simulink model "Quadrotor_14_step4_disc"  (Simulink 7.6)
settings: Solver=ode45  StartTime=0.0  StopTime=200  RelTol=1e-3
undefined symbols (not defined in the file): STARMAC, uav_utilities
libraries: simulink x31, aero_sim_lib x8
(part 1 of 2)
settings Model: Creator=fluffy_bear  LastModifiedBy=jporter
settings OptimizationCC: OptimizeModelRefInitCode=on  LifeSpan=1
settings DebuggingCC: SignalRangeChecking=warning  ParameterDowncastMsg=warning  ParameterOverflowMsg=warning
settings HardwareCC: ProdLargestAtomicInteger=Long  ProdLargestAtomicFloat=Float  ProdEndianess=LittleEndian  ProdHWDeviceType=ARM Compatible->ARM 7
settings SFSimCC: SimParseCustomCode=off
settings RTWCC: SystemTargetFile=ert.tlc  GenCodeOnly=on  TemplateMakefile=ert_default_tmf  Description=Real-Time Workshop Embedded Coder  ProcessScript=ert_make_rtw_hook
settings CodeAppCC: IgnoreCustomStorageClasses=off
settings ERTTargetCC: MultiwordLength=2048  GenerateSampleERTMain=on  CombineSignalStateStructs=on  MultiInstanceERTCode=on  MultiInstanceErrorCode=Warning  ERTCustomFileTemplate=example_file_process.tlc  ConvertIfToSwitch=off

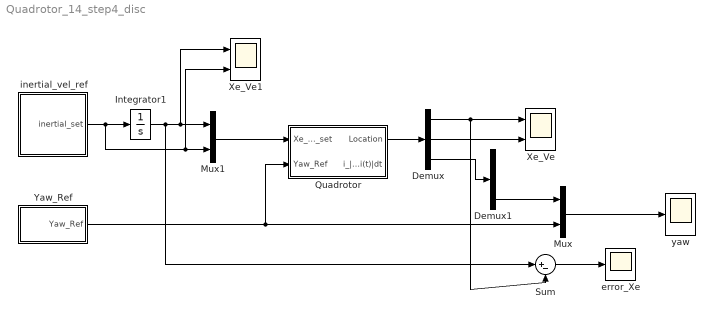
== system Quadrotor_14_step4_disc ==
  Demux : Demux  Outputs=[3,3,3]
  Demux1 : Demux  Outputs=3
  Integrator1 : Integrator
  Mux : Mux  Inputs=2
  Mux1 : Mux  Inputs=2
  Quadrotor : Subsystem  AncestorBlock=uav_utilities/STARMAC
  Sum : Sum  Inputs=|+-
  Xe_Ve : Scope  NumInputPorts=2
      settings: YMin=-25~-1  YMax=35~2.25  MaxDataPoints=100000  SampleInput=on  SampleTime=100/5000
  Xe_Ve1 : Scope  NumInputPorts=2
      settings: YMin=-100~-2  YMax=100~2  SaveName=ScopeData3  MaxDataPoints=100000  SampleInput=on  SampleTime=100/5000
  Yaw_Ref : Subsystem
  error_Xe : Scope
      settings: TimeRange=200  YMin=-1500  YMax=300  SaveName=error_data  MaxDataPoints=20000  Decimation=10  SampleInput=on  SampleTime=100/5000
  inertial_vel_ref : Subsystem
  yaw : Scope
      settings: TimeRange=2  YMin=0  YMax=115000  MaxDataPoints=100000  SampleInput=on  SampleTime=100/5000
  wires:
  inertial_vel_ref/1(inertial_set) -> Integrator1/1, Mux1/2, Xe_Ve1/2
  Yaw_Ref/1(Yaw_Ref) -> Quadrotor/2(Yaw_Ref), Mux/2
  Sum/1 -> error_Xe/1
  Quadrotor/1(Location) -> Demux/1
  Demux/1 -> Sum/2, Xe_Ve/1
  Demux/2 -> Xe_Ve/2
  Mux/1 -> yaw/1
  Demux/3 -> Demux1/1
  Demux1/3 -> Mux/1
  Integrator1/1 -> Sum/1, Mux1/1, Xe_Ve1/1
  Mux1/1 -> Quadrotor/1(Xe_Ve_set)

== system Quadrotor_14_step4_disc/Quadrotor ==
  Xe_Ve_set : Inport  PortDimensions=[6]
  Yaw_Ref : Inport  Port=2  PortDimensions=[1]
  Data Type Conversion : DataTypeConversion  OutDataTypeStr=fixdt(1,32,21)
  Data Type Conversion1 : DataTypeConversion  OutDataTypeStr=fixdt(1,32,29)
  Data Type Conversion2 : DataTypeConversion
  Demux : Demux  Outputs=[3,3]
  GPS : Subsystem
  IMU : Subsystem
  Mux : Mux  Inputs=[3 3 3]
  Rate Transition2 : RateTransition
  Subsystem : Subsystem  MinMaxOverflowLogging=MinMaxAndOverflow
  Term : Terminator
  ZOH : ZeroOrderHold  SampleTime=.01
  ZOH4 : ZeroOrderHold  SampleTime=.01
  Zero-Order Hold : ZeroOrderHold  SampleTime=.02
  dtc : DataTypeConversion
  plant_dynamics : Subsystem  AncestorBlock=aero_sim_lib/starmac_dynamics
  Location : Outport
  i_|P_i(t)|dt : Outport  Port=2
  wires:
  ZOH4/1 -> Data Type Conversion1/1
  Demux/2 -> Term/1
  Demux/1 -> ZOH/1
  Xe_Ve_set/1 -> Demux/1
  Mux/1 -> Location/1
  plant_dynamics/3(euler) -> Mux/3, IMU/1(Euler_c)  "euler"
  plant_dynamics/2(Xe) -> Mux/1, GPS/1(Xe)  "Xe"
  plant_dynamics/1(Ve) -> Mux/2, GPS/2(Ve)  "Ve"
  dtc/1 -> plant_dynamics/1(desired_motor_thrust)
  Zero-Order Hold/1 -> Rate Transition2/1
  Rate Transition2/1 -> dtc/1
  ZOH/1 -> Data Type Conversion/1
  plant_dynamics/5(omega) -> IMU/2(Omega_c)
  plant_dynamics/7(Ab) -> IMU/3(Acc_c)
  plant_dynamics/8(i_|P_i(t)|dt) -> i_|P_i(t)|dt/1
  Yaw_Ref/1 -> ZOH4/1
  IMU/1(Euler_s) -> Subsystem/1(In1)
  IMU/2(Omega_s) -> Subsystem/2(In2)
  IMU/3(Acc_s) -> Subsystem/3(In3)
  GPS/1(Latitude_s) -> Subsystem/4(In4)
  GPS/2(Longitude_s) -> Subsystem/5(In5)
  GPS/3(Height_s) -> Subsystem/6(In6)
  GPS/4(Velocity_xy_s) -> Subsystem/7(In7)
  GPS/5("dot{Height}_s") -> Subsystem/8(In8)
  Data Type Conversion/1 -> Subsystem/9(In9)
  Data Type Conversion1/1 -> Subsystem/10(In10)
  Subsystem/1(Out1) -> Data Type Conversion2/1
  Data Type Conversion2/1 -> Zero-Order Hold/1

== system Quadrotor_14_step4_disc/Yaw_Ref ==
  Signal Generator : SignalGenerator  Frequency=2*.0625*0.25
  Yaw_Ref : Outport
  wires:
  Signal Generator/1 -> Yaw_Ref/1

== system Quadrotor_14_step4_disc/inertial_vel_ref ==
  Signal Generator : SignalGenerator  Amplitude=1.8*[1 -1 -.5]  Frequency=.1*.0625*ones(3,1)
  inertial_set : Outport
  wires:
  Signal Generator/1 -> inertial_set/1

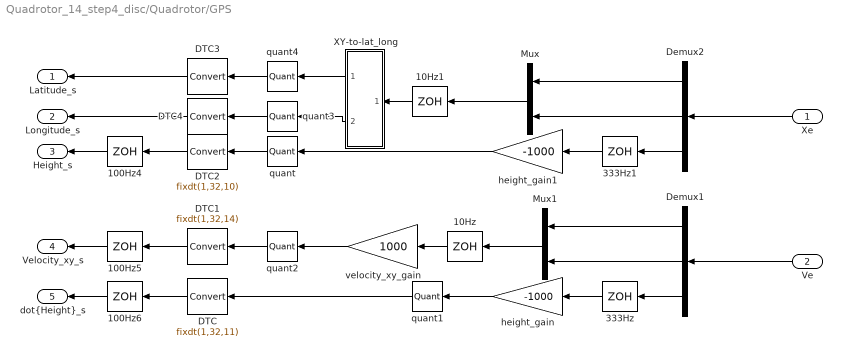
== system Quadrotor_14_step4_disc/Quadrotor/GPS ==
  Xe : Inport
  Ve : Inport  Port=2
  100Hz4 : ZeroOrderHold  SampleTime=.01
  100Hz5 : ZeroOrderHold  SampleTime=.01
  100Hz6 : ZeroOrderHold  SampleTime=.01
  10Hz : ZeroOrderHold  SampleTime=.1
  10Hz1 : ZeroOrderHold  SampleTime=.1
  333Hz : ZeroOrderHold  SampleTime=1/333
  333Hz1 : ZeroOrderHold  SampleTime=1/333
  DTC : DataTypeConversion  OutDataTypeStr=fixdt(1,32,11)
  DTC1 : DataTypeConversion  OutDataTypeStr=fixdt(1,32,14)
  DTC2 : DataTypeConversion  OutDataTypeStr=fixdt(1,32,10)
  DTC3 : DataTypeConversion
  DTC4 : DataTypeConversion
  Demux1 : Demux  Outputs=[1,1,1]
  Demux2 : Demux  Outputs=[1,1,1]
  Mux : Mux  Inputs=2
  Mux1 : Mux  Inputs=2
  XY-to-lat_long : Subsystem  mask{lat_0=36.1658333, lon_0=-86.7844444}
  height_gain : Gain  Gain=-1000  RndMeth=Round  SaturateOnIntegerOverflow=on  OutDataTypeStr=Inherit: Same as input  LockScale=on
  height_gain1 : Gain  Gain=-1000  RndMeth=Round  SaturateOnIntegerOverflow=on  OutDataTypeStr=Inherit: Same as input  LockScale=on
  quant{,1,3..4} (4 alike) : Quantizer  QuantizationInterval=1
  quant2 : Quantizer  QuantizationInterval=ones(2,1)
  velocity_xy_gain : Gain  Gain=1000  RndMeth=Round  SaturateOnIntegerOverflow=on  OutDataTypeStr=Inherit: Same as input  LockScale=on
  Latitude_s : Outport
  Longitude_s : Outport  Port=2
  Height_s : Outport  Port=3
  Velocity_xy_s : Outport  Port=4
  "dot{Height}_s" : Outport  Port=5
  wires:
  Ve/1 -> Demux1/1
  Xe/1 -> Demux2/1
  Demux1/3 -> 333Hz/1
  Demux2/3 -> 333Hz1/1
  Demux2/1 -> Mux/1
  Demux2/2 -> Mux/2
  Demux1/1 -> Mux1/1
  Demux1/2 -> Mux1/2
  333Hz1/1 -> height_gain1/1
  333Hz/1 -> height_gain/1
  Mux1/1 -> 10Hz/1
  10Hz/1 -> velocity_xy_gain/1
  height_gain1/1 -> quant/1
  height_gain/1 -> quant1/1
  quant/1 -> DTC2/1
  quant1/1 -> DTC/1
  velocity_xy_gain/1 -> quant2/1
  quant2/1 -> DTC1/1
  10Hz1/1 -> XY-to-lat_long/1(XY)
  XY-to-lat_long/1(lat) -> quant4/1
  XY-to-lat_long/2(lon) -> quant3/1
  Mux/1 -> 10Hz1/1
  DTC/1 -> 100Hz6/1
  DTC1/1 -> 100Hz5/1
  DTC2/1 -> 100Hz4/1
  DTC3/1 -> Latitude_s/1
  DTC4/1 -> Longitude_s/1
  quant3/1 -> DTC4/1
  quant4/1 -> DTC3/1
  100Hz4/1 -> Height_s/1
  100Hz5/1 -> Velocity_xy_s/1
  100Hz6/1 -> "dot{Height}_s"/1

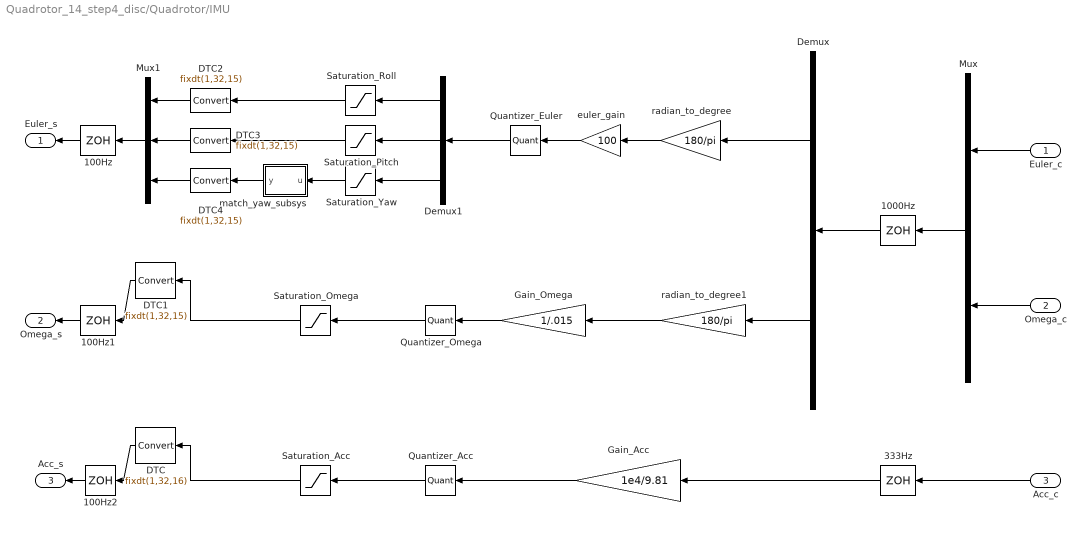
== system Quadrotor_14_step4_disc/Quadrotor/IMU ==
  Euler_c : Inport
  Omega_c : Inport  Port=2
  Acc_c : Inport  Port=3
  1000Hz : ZeroOrderHold  SampleTime=.001
  100Hz : ZeroOrderHold  SampleTime=.01
  100Hz1 : ZeroOrderHold  SampleTime=.01
  100Hz2 : ZeroOrderHold  SampleTime=.01
  333Hz : ZeroOrderHold  SampleTime=1/333
  DTC : DataTypeConversion  OutDataTypeStr=fixdt(1,32,16)
  DTC{1..4} (4 alike) : DataTypeConversion  OutDataTypeStr=fixdt(1,32,15)
  Demux : Demux  Outputs=[3,3]
  Demux1 : Demux  Outputs=[1,1,1]
  Gain_Acc : Gain  Gain=1e4/9.81
  Gain_Omega : Gain  Gain=1/.015
  Mux : Mux  Inputs=[3,3]
  Mux1 : Mux  Inputs=[1,1,1]
  Quantizer_Acc : Quantizer  QuantizationInterval=ones(3,1)
  Quantizer_Euler : Quantizer  QuantizationInterval=ones(3,1)
  Quantizer_Omega : Quantizer  QuantizationInterval=ones(3,1)
  Saturation_Acc : Saturate  UpperLimit=30000  LowerLimit=-30000  RndMeth=Round
      settings: LockScale=on
  Saturation_Omega : Saturate  UpperLimit=((2^15)-1) * ones(3,1)  LowerLimit=-(2^15) * ones(3,1)  OutDataTypeStr=Inherit: Inherit via back propagation  RndMeth=Round
      settings: LockScale=on
  Saturation_Pitch : Saturate  UpperLimit=90*100  LowerLimit=-90*100  RndMeth=Round
      settings: LockScale=on
  Saturation_Roll : Saturate  UpperLimit=90*100  LowerLimit=-90*100  RndMeth=Round
      settings: LockScale=on
  Saturation_Yaw : Saturate  UpperLimit=180*100  LowerLimit=-180*100  RndMeth=Round
      settings: LockScale=on
  euler_gain : Gain  Gain=100
  match_yaw_subsys : Subsystem
  radian_to_degree : Gain  Gain=180/pi
  radian_to_degree1 : Gain  Gain=180/pi
  Euler_s : Outport  LockScale=on
  Omega_s : Outport  Port=2  LockScale=on
  Acc_s : Outport  Port=3  LockScale=on
  wires:
  Mux/1 -> 1000Hz/1
  Euler_c/1 -> Mux/1
  1000Hz/1 -> Demux/1
  Gain_Acc/1 -> Quantizer_Acc/1
  Omega_c/1 -> Mux/2
  333Hz/1 -> Gain_Acc/1
  Saturation_Acc/1 -> DTC/1
  Saturation_Omega/1 -> DTC1/1
  Demux1/1 -> Saturation_Roll/1
  Saturation_Roll/1 -> DTC2/1
  Mux1/1 -> 100Hz/1
  Demux1/2 -> Saturation_Pitch/1
  Saturation_Pitch/1 -> DTC3/1
  Demux1/3 -> Saturation_Yaw/1
  Gain_Omega/1 -> Quantizer_Omega/1
  Demux/1 -> radian_to_degree/1
  radian_to_degree/1 -> euler_gain/1
  Demux/2 -> radian_to_degree1/1
  euler_gain/1 -> Quantizer_Euler/1
  Quantizer_Euler/1 -> Demux1/1
  radian_to_degree1/1 -> Gain_Omega/1
  Quantizer_Omega/1 -> Saturation_Omega/1
  Acc_c/1 -> 333Hz/1
  Quantizer_Acc/1 -> Saturation_Acc/1
  DTC/1 -> 100Hz2/1
  DTC1/1 -> 100Hz1/1
  100Hz/1 -> Euler_s/1
  100Hz1/1 -> Omega_s/1
  100Hz2/1 -> Acc_s/1
  match_yaw_subsys/1(y) -> DTC4/1
  Saturation_Yaw/1 -> match_yaw_subsys/1(u)
  DTC2/1 -> Mux1/1
  DTC3/1 -> Mux1/2
  DTC4/1 -> Mux1/3

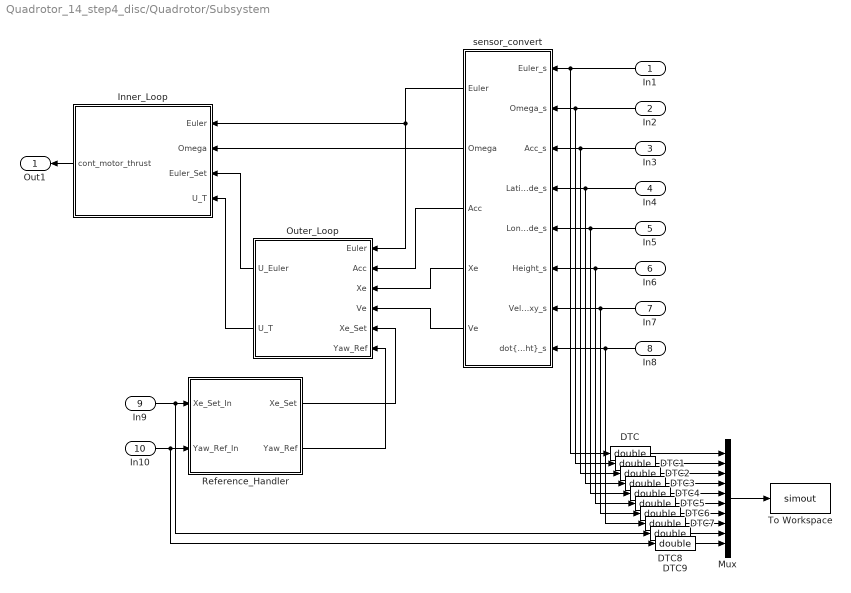
== system Quadrotor_14_step4_disc/Quadrotor/Subsystem ==
  In1 : Inport  OutMin=-36000  OutMax=36000  OutDataTypeStr=fixdt(1,32,15)
  In2 : Inport  Port=2  OutMin=-(2^15)  OutMax=2^15  OutDataTypeStr=fixdt(1,32,15)
  In3 : Inport  Port=3  OutMin=-30000  OutMax=30000  OutDataTypeStr=fixdt(1,32,16)
  In4 : Inport  Port=4  OutMin=-90*1e7  OutMax=90*1e7  OutDataTypeStr=fixdt(1,32,0)
  In5 : Inport  Port=5  OutMin=-180*1e7  OutMax=180*1e7  OutDataTypeStr=fixdt(1,32,0)
  In6 : Inport  Port=6  OutMin=-2000*1000  OutMax=2000*1000  OutDataTypeStr=fixdt(1,32,10)
  In7 : Inport  Port=7  OutMin=-100*1000  OutMax=100*1000  OutDataTypeStr=fixdt(1,32,14)
  In8 : Inport  Port=8  OutMin=-100*1000  OutMax=1000*1000  OutDataTypeStr=fixdt(1,32,11)
  In9 : Inport  Port=9  OutMin=-1000  OutMax=1000  OutDataTypeStr=fixdt(1,32,21)
  In10 : Inport  Port=10  OutMin=-pi  OutMax=pi  OutDataTypeStr=fixdt(1,32,29)
  DTC{,1..9} (10 alike) : DataTypeConversion  OutDataTypeStr=double
  Inner_Loop : Subsystem
  Mux : Mux  Inputs=10
  Outer_Loop : Subsystem
  Reference_Handler : Subsystem
  To Workspace : ToWorkspace  VariableName=simout  SampleTime=-1  SaveFormat=Structure
  sensor_convert : Subsystem
  Out1 : Outport
  wires:
  Outer_Loop/1(U_Euler) -> Inner_Loop/3(Euler_Set)
  Outer_Loop/2(U_T) -> Inner_Loop/4(U_T)
  sensor_convert/1(Euler) -> Inner_Loop/1(Euler), Outer_Loop/1(Euler)
  sensor_convert/2(Omega) -> Inner_Loop/2(Omega)
  sensor_convert/3(Acc) -> Outer_Loop/2(Acc)
  sensor_convert/4(Xe) -> Outer_Loop/3(Xe)
  sensor_convert/5(Ve) -> Outer_Loop/4(Ve)
  Reference_Handler/1(Xe_Set) -> Outer_Loop/5(Xe_Set)
  Reference_Handler/2(Yaw_Ref) -> Outer_Loop/6(Yaw_Ref)
  In1/1 -> sensor_convert/1(Euler_s), DTC/1
  In2/1 -> sensor_convert/2(Omega_s), DTC1/1
  In3/1 -> sensor_convert/3(Acc_s), DTC2/1
  Inner_Loop/1(cont_motor_thrust) -> Out1/1
  In4/1 -> sensor_convert/4(Latitude_s), DTC3/1
  In5/1 -> sensor_convert/5(Longitude_s), DTC4/1
  In6/1 -> sensor_convert/6(Height_s), DTC5/1
  In7/1 -> sensor_convert/7(Velocity_xy_s), DTC6/1
  In8/1 -> sensor_convert/8("dot{Height}_s"), DTC7/1
  In9/1 -> Reference_Handler/1(Xe_Set_In), DTC8/1
  In10/1 -> Reference_Handler/2(Yaw_Ref_In), DTC9/1
  Mux/1 -> To Workspace/1
  DTC/1 -> Mux/1
  DTC1/1 -> Mux/2
  DTC2/1 -> Mux/3
  DTC3/1 -> Mux/4
  DTC4/1 -> Mux/5
  DTC5/1 -> Mux/6
  DTC6/1 -> Mux/7
  DTC7/1 -> Mux/8
  DTC8/1 -> Mux/9
  DTC9/1 -> Mux/10

== system Quadrotor_14_step4_disc/Quadrotor/plant_dynamics ==
  desired_motor_thrust : Inport
  6DOF_Euler_Angles : Subsystem  AncestorBlock=aero_sim_lib/6DOF (Euler Angles)_CMU  mask{XYZe_0=[0.01;0.01;0], Vb_0=[0;0;0], euler_0=[0;0;0], omega_0=[0;0;0], M=1.8623, I=diag([0.02759 0.02771 0.04806])}
      mask prompts: XYZe_0 "Initial position in inertial axes [Xe,Ye,Ze]:"; Vb_0 "Initial velocity in body axes [U,v,w]:"; euler_0 "Initial Euler orientation [roll, pitch, yaw]=[phi,theta,psi]:"; omega_0 "Initial body rotation rates [p,q,r]=omega:"; M "Initial mass:"; I "Inertial:"
  Abs : Abs
  Dot Product : DotProduct  InputSameDT=on  OutDataTypeStr=Inherit: Inherit via internal rule
  Integrator : Integrator
  Product : Product  Multiplication=Matrix(*)  RndMeth=Zero
  Product1 : Product  Multiplication=Matrix(*)  RndMeth=Zero
  Sum : Sum  Inputs=|+++
  Sum1 : Sum  Inputs=|+-
  Viscous Drag : Gain  Gain=-.1
  gravity_effects : Constant  Value=1.8623*[0;0;9.8]
  gravity_effects1 : Constant  Value=zeros(3,1)
  starmac_blade_flapping_effects : Subsystem  AncestorBlock=aero_sim_lib/starmac_blade_flapping_effects
  starmac_motor_dynamics : Subsystem  AncestorBlock=aero_sim_lib/starmac_motor_dynamics  mask{tau_motor=.1, T_nom=1.8263*9.8/4, thrust_max=9.8, thrust_min=0, motor_lag_enable=on, motor_variance=.01*(.05*9.8/4)^2, Ts=1/76}
      mask prompts: tau_motor "tau_motor (seconds):"; T_nom "nominal thrust (N):"; thrust_max "maximum thrust (N):"; thrust_min "minimum thrust (N):"; motor_lag_enable "Motor Lag Enabled:"; motor_variance "Motor Variance [motor_variance]:"; Ts "Motor Update Rate (seconds):"
  Ve : Outport
  Xe : Outport  Port=2
  euler : Outport  Port=3
  DCM : Outport  Port=4
  omega : Outport  Port=5
  domega/dt : Outport  Port=6
  Ab : Outport  Port=7
  i_|P_i(t)|dt : Outport  Port=8
  wires:
  desired_motor_thrust/1 -> starmac_motor_dynamics/1(desired_motor_thrust)
  starmac_blade_flapping_effects/1(body_forces) -> Sum/2, Dot Product/1
  starmac_blade_flapping_effects/2(body_moments) -> 6DOF_Euler_Angles/2(M_xyz(Nm))
  Viscous Drag/1 -> Sum/3
  6DOF_Euler_Angles/5(Vb) -> Sum1/1, Dot Product/2
  Product1/1 -> Sum1/2
  Sum1/1 -> Viscous Drag/1, starmac_blade_flapping_effects/2(v_body_relative)
  gravity_effects/1 -> Product/2
  6DOF_Euler_Angles/4(DCM) -> Product1/1, Product/1, DCM/1
  Sum/1 -> 6DOF_Euler_Angles/1(F_xyz(N))
  Product/1 -> Sum/1
  starmac_motor_dynamics/1(motor_thrust) -> starmac_blade_flapping_effects/1(motor_thrusts)
  6DOF_Euler_Angles/1(Ve) -> Ve/1
  6DOF_Euler_Angles/2(Xe) -> Xe/1
  6DOF_Euler_Angles/3(euler) -> euler/1
  6DOF_Euler_Angles/6(omega) -> omega/1
  6DOF_Euler_Angles/7(domega/dt) -> domega/dt/1
  6DOF_Euler_Angles/8(Ab) -> Ab/1
  Integrator/1 -> i_|P_i(t)|dt/1
  Dot Product/1 -> Abs/1
  Abs/1 -> Integrator/1
  gravity_effects1/1 -> Product1/2

== system Quadrotor_14_step4_disc/Quadrotor/GPS/XY-to-lat_long ==
  XY : Inport
  XY-to-lat_long : Stateflow chart  TreatAsAtomicUnit=on
  lat : Outport
  lon : Outport  Port=2
  wires:
  XY-to-lat_long/1(lat) -> lat/1
  XY/1 -> XY-to-lat_long/1(XY)
  XY-to-lat_long/2(lon) -> lon/1

== system Quadrotor_14_step4_disc/Quadrotor/IMU/match_yaw_subsys ==
  u : Inport
  Constant : Constant  Value=360
  Sum : Sum  Inputs=++|
  Switch : Switch
  euler_gain1 : Gain  Gain=100
  y : Outport
  wires:
  u/1 -> Switch/2, Sum/1, Switch/1
  Constant/1 -> euler_gain1/1
  euler_gain1/1 -> Sum/2
  Sum/1 -> Switch/3
  Switch/1 -> y/1

== system Quadrotor_14_step4_disc/Quadrotor/Subsystem/Inner_Loop ==
  Euler : Inport
  Omega : Inport  Port=2
  Euler_Set : Inport  Port=3
  U_T : Inport  Port=4
  DTC{,1..3} (4 alike) : DataTypeConversion
  euler_controller : Subsystem  mask{K=1, K_e=7.5/.65, K_o=.5}
      mask prompts: K "Loop Gain [K]:"; K_e "Euler Gain [K_e]:"; K_o "Omega Gain [K_o]:"
  lead_motor : Subsystem  mask{tau_motor=.10, t_s=.01}
      mask init:
      | Hs=tf([tau_motor 1],[t_s/pi 1]);
      | Hz=ipesh_transform(Hs,t_s);
  thrust_limit : Saturate  UpperLimit=10*ones(4,1)  LowerLimit=0*ones(4,1)  OutDataTypeStr=fixdt(1,32,27)
  u_T_u_torque_motor_thrust : Subsystem  mask{dx=.3048, K_torque=.47}
      mask prompts: dx "X distance of motor from CG [dx](meters):"; K_torque "Ktorque [K_torque]:"
      mask init:
      | M=[0 -dx 0 dx;
      |    dx 0 -dx 0;
      |    -K_torque K_torque -K_torque K_torque;
      |    1 1 1 1];
      | Mi=inv(M);
  cont_motor_thrust : Outport
  wires:
  Euler_Set/1 -> DTC/1
  U_T/1 -> DTC3/1
  euler_controller/1(u_torque) -> u_T_u_torque_motor_thrust/1(u_torque)
  thrust_limit/1 -> cont_motor_thrust/1
  u_T_u_torque_motor_thrust/1(cont_motor_thrust) -> lead_motor/1(thrust_in)
  lead_motor/1(thrust_out) -> thrust_limit/1
  Euler/1 -> DTC1/1
  Omega/1 -> DTC2/1
  DTC/1 -> euler_controller/1(euler_set)
  DTC1/1 -> euler_controller/2(euler)
  DTC2/1 -> euler_controller/3(omega)
  DTC3/1 -> u_T_u_torque_motor_thrust/2(u_T)

== system Quadrotor_14_step4_disc/Quadrotor/Subsystem/Outer_Loop ==
  Euler : Inport  PortDimensions=[3]
  Acc : Inport  Port=2  PortDimensions=[3]
  Xe : Inport  Port=3  PortDimensions=[3]
  Ve : Inport  Port=4  PortDimensions=[3]
  Xe_Set : Inport  Port=5  PortDimensions=[3]
  Yaw_Ref : Inport  Port=6  PortDimensions=[1]
  DTC : DataTypeConversion
  DTC1 : DataTypeConversion  OutDataTypeStr=fixdt(1,32,26)
  DTC2 : DataTypeConversion  OutDataTypeStr=fixdt(1,32,27)
  DTC3 : DataTypeConversion  OutDataTypeStr=fixdt(1,32,20)
  DTC4 : DataTypeConversion
  DTC5 : DataTypeConversion
  Demux : Demux  Outputs=3
  body_to_inertial : Subsystem
  inertial_pos_controller : Subsystem
  rate_limiter_quant : Subsystem  mask{wn=2*pi, zeta=0.9, Vmax=2, T=0.01}
      mask prompts: wn "omega_n"; Vmax "Max velocity"; T "Sample time"
      mask init:
      | Hs=tf([wn^2],[1,2*zeta*wn,wn^2]);
      | Hz=ipesh_transform(Hs,T);
  sensor_fusion : Subsystem  mask{tau=.1, Ts=.01, Ts_gps=.1}
      mask prompts: tau "low-pass time constant (sec) [tau]"; Ts "Sample time [Ts]"; Ts_gps "GPS Sample Time [Ts_gps]"
  U_Euler : Outport  PortDimensions=[3]
  U_T : Outport  Port=2  PortDimensions=[1]
  wires:
  Xe_Set/1 -> DTC3/1
  inertial_pos_controller/1(u_T) -> U_T/1
  inertial_pos_controller/2(u_euler) -> U_Euler/1
  Euler/1 -> DTC2/1
  Acc/1 -> DTC1/1
  sensor_fusion/1(Xe) -> inertial_pos_controller/2(Xe)
  sensor_fusion/2(Ve) -> inertial_pos_controller/3(Ve)
  body_to_inertial/1(Xe) -> sensor_fusion/1(Xe_f)
  body_to_inertial/2(Ve) -> sensor_fusion/2(Ve_f)
  Xe/1 -> DTC4/1
  Ve/1 -> DTC5/1
  rate_limiter_quant/1(Xr_set) -> inertial_pos_controller/1(Xe_set)
  Demux/3 -> inertial_pos_controller/4(Yaw_actual)
  Yaw_Ref/1 -> DTC/1
  DTC/1 -> inertial_pos_controller/5(Yaw_set)
  DTC1/1 -> body_to_inertial/2(Ab)
  DTC2/1 -> body_to_inertial/1(euler), Demux/1
  DTC3/1 -> rate_limiter_quant/1(Xe_set)
  DTC4/1 -> sensor_fusion/3(Xe_s)
  DTC5/1 -> sensor_fusion/4(Ve_s)

== system Quadrotor_14_step4_disc/Quadrotor/Subsystem/Reference_Handler ==
  Xe_Set_In : Inport
  Yaw_Ref_In : Inport  Port=2
  DTC : DataTypeConversion
  DTC1 : DataTypeConversion
  Gain : Gain  ParamMin=1  ParamMax=1  OutDataTypeStr=fixdt(1,32,21)
  Gain1 : Gain  ParamMin=1  ParamMax=1  OutDataTypeStr=fixdt(1,32,29)
  Xe_Set : Outport
  Yaw_Ref : Outport  Port=2
  wires:
  Xe_Set_In/1 -> Gain/1
  Yaw_Ref_In/1 -> Gain1/1
  Gain1/1 -> DTC1/1
  Gain/1 -> DTC/1
  DTC/1 -> Xe_Set/1
  DTC1/1 -> Yaw_Ref/1

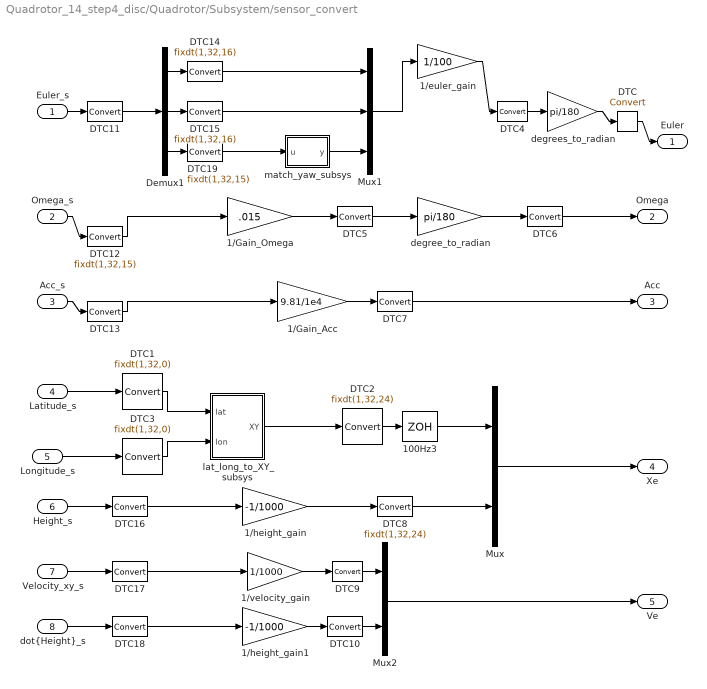
== system Quadrotor_14_step4_disc/Quadrotor/Subsystem/sensor_convert ==
  Euler_s : Inport
  Omega_s : Inport  Port=2
  Acc_s : Inport  Port=3
  Latitude_s : Inport  Port=4
  Longitude_s : Inport  Port=5
  Height_s : Inport  Port=6
  Velocity_xy_s : Inport  Port=7
  "dot{Height}_s" : Inport  Port=8
  1/Gain_Acc : Gain  Gain=9.81/1e4  ParamMin=9.81/1e4  ParamMax=9.81/1e4  OutDataTypeStr=fixdt(1,32,26)
  1/Gain_Omega : Gain  Gain=.015  ParamMin=.015  ParamMax=.015  OutDataTypeStr=fixdt(1,32,22)
  1/euler_gain : Gain  Gain=1/100  ParamMin=1/100  ParamMax=1/100  OutDataTypeStr=fixdt(1,32,23)
  1/height_gain : Gain  Gain=-1/1000  ParamMin=-1/1000  ParamMax=-1/1000  OutDataTypeStr=fixdt(1,32,25)
  1/height_gain1 : Gain  Gain=-1/1000  ParamMin=-1/1000  ParamMax=-1/1000  OutDataTypeStr=fixdt(1,32,31)
  1/velocity_gain : Gain  Gain=1/1000  ParamMin=1/1000  ParamMax=1/1000  OutDataTypeStr=fixdt(1,32,30)
  100Hz3 : ZeroOrderHold  SampleTime=.01
  DTC{,4..7,9..11,13,16..18} (12 alike) : DataTypeConversion
  DTC1 : DataTypeConversion  OutDataTypeStr=fixdt(1,32,0)
  DTC12 : DataTypeConversion  OutDataTypeStr=fixdt(1,32,15)
  DTC14 : DataTypeConversion  OutMin=-9000  OutMax=9000  OutDataTypeStr=fixdt(1,32,16)
  DTC15 : DataTypeConversion  OutMin=-9000  OutMax=9000  OutDataTypeStr=fixdt(1,32,16)
  DTC19 : DataTypeConversion  OutMin=0  OutMax=36000  OutDataTypeStr=fixdt(1,32,15)
  DTC2 : DataTypeConversion  OutDataTypeStr=fixdt(1,32,24)
  DTC3 : DataTypeConversion  OutDataTypeStr=fixdt(1,32,0)
  DTC8 : DataTypeConversion  OutDataTypeStr=fixdt(1,32,24)
  Demux1 : Demux  Outputs=3
  Mux : Mux  Inputs=[2,1]
  Mux1 : Mux  Inputs=3
  Mux2 : Mux  Inputs=[2,1]
  degree_to_radian : Gain  Gain=pi/180  ParamMin=pi/180  ParamMax=pi/180  OutDataTypeStr=fixdt(1,32,27)
  degrees_to_radian : Gain  Gain=pi/180  ParamMin=pi/180  ParamMax=pi/180  OutDataTypeStr=fixdt(1,32,27)
  lat_long_to_XY_subsys : Subsystem
  match_yaw_subsys : Subsystem
  Euler : Outport
  Omega : Outport  Port=2
  Acc : Outport  Port=3
  Xe : Outport  Port=4
  Ve : Outport  Port=5
  wires:
  Omega_s/1 -> DTC12/1
  1/Gain_Omega/1 -> DTC5/1
  1/Gain_Acc/1 -> DTC7/1
  Acc_s/1 -> DTC13/1
  degree_to_radian/1 -> DTC6/1
  Euler_s/1 -> DTC11/1
  Mux1/1 -> 1/euler_gain/1
  degrees_to_radian/1 -> DTC/1
  1/euler_gain/1 -> DTC4/1
  Demux1/1 -> DTC14/1
  Demux1/2 -> DTC15/1
  match_yaw_subsys/1(y) -> Mux1/3
  Demux1/3 -> DTC19/1
  Velocity_xy_s/1 -> DTC17/1
  Height_s/1 -> DTC16/1
  1/height_gain/1 -> DTC8/1
  Latitude_s/1 -> DTC1/1
  Longitude_s/1 -> DTC3/1
  lat_long_to_XY_subsys/1(XY) -> DTC2/1
  100Hz3/1 -> Mux/1
  Mux/1 -> Xe/1
  "dot{Height}_s"/1 -> DTC18/1
  1/height_gain1/1 -> DTC10/1
  Mux2/1 -> Ve/1
  DTC2/1 -> 100Hz3/1
  1/velocity_gain/1 -> DTC9/1
  DTC1/1 -> lat_long_to_XY_subsys/1(lat)
  DTC3/1 -> lat_long_to_XY_subsys/2(lon)
  DTC/1 -> Euler/1
  DTC4/1 -> degrees_to_radian/1
  DTC5/1 -> degree_to_radian/1
  DTC6/1 -> Omega/1
  DTC7/1 -> Acc/1
  DTC8/1 -> Mux/2
  DTC9/1 -> Mux2/1
  DTC10/1 -> Mux2/2
  DTC11/1 -> Demux1/1
  DTC12/1 -> 1/Gain_Omega/1
  DTC13/1 -> 1/Gain_Acc/1
  DTC16/1 -> 1/height_gain/1
  DTC17/1 -> 1/velocity_gain/1
  DTC18/1 -> 1/height_gain1/1
  DTC14/1 -> Mux1/1
  DTC15/1 -> Mux1/2
  DTC19/1 -> match_yaw_subsys/1(u)

== system Quadrotor_14_step4_disc/Quadrotor/plant_dynamics/6DOF_Euler_Angles ==
  note: This subsystem models a 6 degree of freedom (6DOF) system in Euler angles.
      | A Direct Cosine Matrix (DCM) is produced to allow for easy transformations to
      | and from the reference frame of the body.  Enter appropriate Parameters in the dialog menu.
      | Follows Euler Angle Sequence (1,2,3), see Section 5.6, Representing Attitude: Euler Angles, Unit
      | Quaternions, and Rotation by James Diebel.  Interface matches that from the Aerospace Toolbox
      | for non variable mass (6DoF EoM (Body Axis) for Euler Angles).
      |
      | J. Kapinski
      | Carnegia Mellon University
      | 7/2007
      | Revised:
      | Nicholas Kottenstette, ISIS, 8/2008
  note: 6 DOF System Model
  F_xyz(N) : Inport
  M_xyz(Nm) : Inport  Port=2  PortDimensions=3
  body_euler_to_earth : aero_sim_lib/body_euler_to_earth  SystemSampleTime=-1  XYZe_0=XYZe_0
  continuous_body_dynamics : aero_sim_lib/continuous_body_dynamics  SystemSampleTime=-1  M=M  Vb_0=Vb_0
  continuous_inertia_body_dynamics : aero_sim_lib/continuous_inertia_body_dynamics  SystemSampleTime=-1  I=I  omega_0=omega_0
  omega_to_euler : aero_sim_lib/omega_to_euler  SystemSampleTime=-1  euler_0=euler_0
  Ve : Outport
  Xe : Outport  Port=2
  euler : Outport  Port=3
  DCM : Outport  Port=4
  Vb : Outport  Port=5
  omega : Outport  Port=6
  domega/dt : Outport  Port=7
  Ab : Outport  Port=8
  wires:
  body_euler_to_earth/3 -> Xe/1
  body_euler_to_earth/2 -> DCM/1
  body_euler_to_earth/1 -> Ve/1
  omega_to_euler/1 -> body_euler_to_earth/1, euler/1
  continuous_inertia_body_dynamics/2 -> domega/dt/1
  continuous_body_dynamics/2 -> Ab/1
  continuous_body_dynamics/1 -> body_euler_to_earth/2, Vb/1
  continuous_inertia_body_dynamics/1 -> omega_to_euler/1, continuous_body_dynamics/2, omega/1
  F_xyz(N)/1 -> continuous_body_dynamics/1
  M_xyz(Nm)/1 -> continuous_inertia_body_dynamics/1

== system Quadrotor_14_step4_disc/Quadrotor/plant_dynamics/starmac_blade_flapping_effects ==
  motor_thrusts : Inport
  v_body_relative : Inport  Port=2
  Pick First 2 Elements : Constant  Value=[1 0 0; 0 1 0; 0 0 0]
  Product : Product  RndMeth=Zero
  Product2 : Product  Multiplication=Matrix(*)  RndMeth=Zero
  Product4 : Product  RndMeth=Zero
  Sum : Sum  Inputs=|++
  Sum of Elements : Sum  Inputs=+
  starmac_body_moments : Subsystem  AncestorBlock=aero_sim_lib/starmac_body_moments  mask{dx=.3048, dz=.07, K_torque=.47}
  starmac_flapping_dynamics : Subsystem  AncestorBlock=aero_sim_lib/starmac_flapping_dynamics  mask{K_a1s=.009, K_beta=.23}
  starmac_vertical_effect_dynamics : Subsystem  AncestorBlock=aero_sim_lib/starmac_vertical_effect_dynamics  mask{tau_motor=0.1, R=0.127, Alpha=(pi/180)*[-85:5:85], Vinf=[0:0.5:6], Thrust=9.8*[0.3:0.02:0.8]}
      mask prompts: tau_motor "motor time constant (s)"; R "radius of propeller (m)"; Alpha "Alpha (radians)"; Vinf "Vinf (radians)"; Thrust "Propeller Thrust (N)"
      mask init:
      | rho = 1.2;
      | A = pi*R^2;
      | Vh = sqrt(Thrust/(2*rho*A));
      | for i = 1:length(Vh)
      |     for j = 1:length(Vinf)
      |         for k = 1:length(Alpha)
      |             Vi(k,j,i) = find_vi(Vh(i),Vinf(j),Alpha(k));
      |             ToverTh(k,j,i) = min(10,max(0.1,Vh(i)/(Vi(k,j,i)+Vinf(j)*sin(Alpha(k)))));
      |         end
      |     end
      | end
  body_forces : Outport
  body_moments : Outport  Port=2
  wires:
  starmac_flapping_dynamics/2(rotor_blade_moments) -> Sum/2
  Sum/1 -> body_moments/1
  starmac_body_moments/1(Body Moments) -> Sum/1
  starmac_flapping_dynamics/1(thrust_vector) -> Product4/2, starmac_body_moments/2(Thrust Vector)
  Product4/1 -> body_forces/1
  Sum of Elements/1 -> Product4/1
  Product2/1 -> starmac_flapping_dynamics/1(Vb2_hat)
  v_body_relative/1 -> Product2/2, starmac_vertical_effect_dynamics/2(v_body_relative)
  Pick First 2 Elements/1 -> Product2/1
  motor_thrusts/1 -> Product/1, starmac_vertical_effect_dynamics/1(motor_thrusts)
  starmac_vertical_effect_dynamics/1(thrust_multiplier) -> Product/2
  Product/1 -> Sum of Elements/1, starmac_body_moments/1(Thrust Magnitudes)

== system Quadrotor_14_step4_disc/Quadrotor/plant_dynamics/starmac_motor_dynamics ==
  desired_motor_thrust : Inport
  Band-Limited White Noise : simulink/Sources/Band-Limited White Noise  SystemSampleTime=-1  Cov=Ts*motor_variance*ones(4,1)  Ts=Ts  seed=22341+[0 1 2 3]'
  Constant : Constant  Value=motor_lag_enable
  Saturation : Saturate  UpperLimit=thrust_max*ones(4,1)  LowerLimit=thrust_min*ones(4,1)
  State-Space : StateSpace  A=-(1/tau_motor)*eye(4)  B=(1/tau_motor)*eye(4)  C=eye(4)  D=zeros(4,4)  X0=T_nom*ones(4,1)
  Sum : Sum  Inputs=|++
  Switch : Switch  Criteria=u2 > Threshold
  motor_thrust : Outport
  wires:
  desired_motor_thrust/1 -> State-Space/1, Switch/3
  Sum/1 -> motor_thrust/1
  Saturation/1 -> Sum/1
  Band-Limited White Noise/1 -> Sum/2
  State-Space/1 -> Switch/1
  Switch/1 -> Saturation/1
  Constant/1 -> Switch/2

== system Quadrotor_14_step4_disc/Quadrotor/Subsystem/Inner_Loop/euler_controller ==
  euler_set : Inport
  euler : Inport  Port=2
  omega : Inport  Port=3
  DTC : DataTypeConversion
  DTC1 : DataTypeConversion
  K_euler : Gain  Gain=K_e
  K_omega : Gain  Gain=K_o
  Sum : Sum  Inputs=|+-
  Sum1 : Sum  Inputs=|+-
  torque_limit : Saturate  UpperLimit=9.8*.3048*ones(3,1)  LowerLimit=-9.8*.3048*ones(3,1)  OutDataTypeStr=Inherit: Inherit via back propagation
  u_torque : Outport
  wires:
  Sum/1 -> K_omega/1
  euler_set/1 -> Sum1/1  "euler_set"
  Sum1/1 -> K_euler/1
  euler/1 -> Sum1/2  "euler"
  K_euler/1 -> DTC/1  "u_omega"
  torque_limit/1 -> u_torque/1
  K_omega/1 -> DTC1/1
  omega/1 -> Sum/2  "omega"
  DTC/1 -> Sum/1
  DTC1/1 -> torque_limit/1

== system Quadrotor_14_step4_disc/Quadrotor/Subsystem/Inner_Loop/lead_motor ==
  thrust_in : Inport
  DTC{,1..3} (4 alike) : DataTypeConversion
  Demux : Demux
  Discrete Transfer Fcn{,1..3} (4 alike) : DiscreteTransferFcn  Numerator=Hz.num{1}  Denominator=Hz.den{1}  SampleTime=-1
  Mux : Mux
  thrust_out : Outport
  wires:
  thrust_in/1 -> Demux/1  "x"
  Demux/1 -> Discrete Transfer Fcn/1
  Demux/2 -> Discrete Transfer Fcn1/1
  Demux/3 -> Discrete Transfer Fcn2/1
  Mux/1 -> thrust_out/1
  Discrete Transfer Fcn/1 -> DTC3/1
  Discrete Transfer Fcn1/1 -> DTC2/1
  Discrete Transfer Fcn2/1 -> DTC1/1
  Demux/4 -> Discrete Transfer Fcn3/1
  Discrete Transfer Fcn3/1 -> DTC/1
  DTC/1 -> Mux/4
  DTC1/1 -> Mux/3
  DTC2/1 -> Mux/2
  DTC3/1 -> Mux/1

== system Quadrotor_14_step4_disc/Quadrotor/Subsystem/Inner_Loop/u_T_u_torque_motor_thrust ==
  u_torque : Inport
  u_T : Inport  Port=2
  DTC : DataTypeConversion
  Mi : Gain  Gain=Mi  Multiplication=Matrix(K*u)
  Mux : Mux  Inputs=2
  cont_motor_thrust : Outport
  wires:
  u_torque/1 -> Mux/1
  u_T/1 -> Mux/2
  Mi/1 -> DTC/1
  Mux/1 -> Mi/1
  DTC/1 -> cont_motor_thrust/1

== system Quadrotor_14_step4_disc/Quadrotor/Subsystem/Outer_Loop/body_to_inertial ==
  euler : Inport
  Ab : Inport  Port=2
  Ab_to_Ae_subsys : Subsystem
  Ab_to_Ae_subsys_quant : Subsystem
  inertial_vel_and pos_est : Subsystem  mask{Ts=.01}
      mask prompts: Ts "Sample Time [Ts] (seconds):"
  Xe : Outport
  Ve : Outport  Port=2
  wires:
  euler/1 -> Ab_to_Ae_subsys_quant/1(euler1)
  Ab/1 -> Ab_to_Ae_subsys_quant/2(Ab)
  Ab_to_Ae_subsys_quant/1(Ae) -> inertial_vel_and pos_est/1(Ab)
  inertial_vel_and pos_est/1(Vb) -> Ve/1
  inertial_vel_and pos_est/2(Xb) -> Xe/1

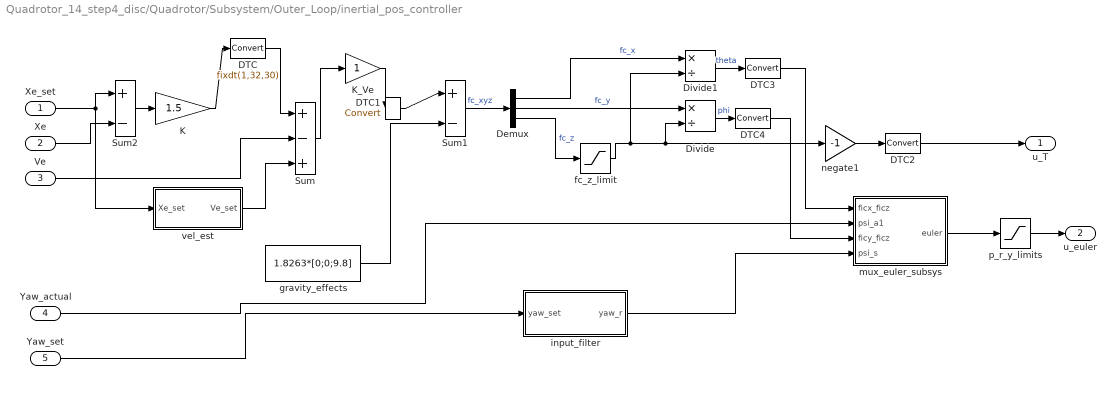
== system Quadrotor_14_step4_disc/Quadrotor/Subsystem/Outer_Loop/inertial_pos_controller ==
  Xe_set : Inport
  Xe : Inport  Port=2
  Ve : Inport  Port=3
  Yaw_actual : Inport  Port=4
  Yaw_set : Inport  Port=5
  DTC : DataTypeConversion  OutDataTypeStr=fixdt(1,32,30)
  DTC{1..4} (4 alike) : DataTypeConversion
  Demux : Demux  Outputs=3
  Divide : Product  Inputs=*/  OutDataTypeStr=fixdt(1,32,35)
  Divide1 : Product  Inputs=*/  OutDataTypeStr=fixdt(1,32,35)
  K : Gain  Gain=1.5  ParamMin=0  ParamMax=30  OutDataTypeStr=fixdt(1,32,30)
  K_Ve : Gain  ParamMin=0  ParamMax=30  OutDataTypeStr=fixdt(1,32,30)
  Sum : Sum  Inputs=|+-+  OutDataTypeStr=fixdt(1,32,30)
  Sum1 : Sum  Inputs=|+-  OutDataTypeStr=fixdt(1,32,26)
  Sum2 : Sum  Inputs=|+-  OutDataTypeStr=fixdt(1,32,30)
  fc_z_limit : Saturate  UpperLimit=-(1/8)*9.81  LowerLimit=-4*9.81  OutDataTypeStr=fixdt(1,32,25)
  gravity_effects : Constant  Value=1.8263*[0;0;9.8]  OutMin=0  OutMax=(1.8263*9.8)+2^-18  OutDataTypeStr=fixdt(1,32,26)
  input_filter : Subsystem  mask{wn=1, zeta=0.9, T=0.01}
      mask prompts: wn "omega_n"; T "Sample time"
      mask init:
      | Hs=tf([wn^2],[1,2*zeta*wn,wn^2]);
      | Hz=ipesh_transform(Hs,T);
  mux_euler_subsys : Subsystem
  negate1 : Gain  Gain=-1  ParamMin=-1  ParamMax=-1  OutDataTypeStr=fixdt(1,32,26)
  p_r_y_limits : Saturate  UpperLimit=[pi/4,pi/4,inf]  LowerLimit=-[pi/4,pi/4,inf]  OutDataTypeStr=fixdt(1,32,28)
  vel_est : Subsystem  mask{tau_f=.01/pi, T=.01}
      mask prompts: T "sample rate"
      mask init:
      | Hs=tf([1 0],[T/pi 1]);
      | Hz=ipesh_transform(Hs,T);
  u_T : Outport
  u_euler : Outport  Port=2
  wires:
  fc_z_limit/1 -> Divide1/2, Divide/2, negate1/1
  Xe_set/1 -> Sum2/1, vel_est/1(Xe_set)
  negate1/1 -> DTC2/1
  p_r_y_limits/1 -> u_euler/1
  Demux/1 -> Divide1/1  "fc_x"
  Demux/3 -> fc_z_limit/1  "fc_z"
  mux_euler_subsys/1(euler) -> p_r_y_limits/1
  Sum1/1 -> Demux/1  "fc_xyz"
  gravity_effects/1 -> Sum1/2
  Sum/1 -> K_Ve/1
  Xe/1 -> Sum2/2
  Sum2/1 -> K/1
  K/1 -> DTC/1
  Demux/2 -> Divide/1  "fc_y"
  K_Ve/1 -> DTC1/1
  Ve/1 -> Sum/2
  vel_est/1(Ve_set) -> Sum/3
  Divide1/1 -> DTC3/1  "theta"
  Divide/1 -> DTC4/1  "phi"
  input_filter/1(yaw_r) -> mux_euler_subsys/4(psi_s)
  Yaw_set/1 -> input_filter/1(yaw_set)
  DTC/1 -> Sum/1
  DTC1/1 -> Sum1/1
  DTC2/1 -> u_T/1
  DTC3/1 -> mux_euler_subsys/1(ficx_ficz)
  Yaw_actual/1 -> mux_euler_subsys/2(psi_a1)
  DTC4/1 -> mux_euler_subsys/3(ficy_ficz)

== system Quadrotor_14_step4_disc/Quadrotor/Subsystem/Outer_Loop/rate_limiter_quant ==
  Xe_set : Inport
  Constant : Constant  Value=T  OutDataTypeStr=fixdt(1,32,32)
  Constant1 : Constant  Value=Vmax  OutDataTypeStr=fixdt(1,32,27)
  DTC : DataTypeConversion  OutDataTypeStr=fixdt(1,32,20)
  DTC1 : DataTypeConversion
  DTC2 : DataTypeConversion
  Demux : Demux  Outputs=3
  Discrete Transfer Fcn3 : DiscreteTransferFcn  Numerator=Hz.num{1}  Denominator=Hz.den{1}  SampleTime=-1  StateDataTypeStr=fixdt(1,64,29)  NumCoefDataTypeStr=fixdt(1,64,39)  DenCoefDataTypeStr=fixdt(1,64,29)  NumProductDataTypeStr=fixdt(1,64,39)  DenProductDataTypeStr=fixdt(1,64,29)  NumAccumDataTypeStr=fixdt(1,64,35)  DenAccumDataTypeStr=fixdt(1,64,25)  OutDataTypeStr=fixdt(1,64,20)  RndMeth=Nearest  SaturateOnIntegerOverflow=on
  Discrete Transfer Fcn4 : DiscreteTransferFcn  Numerator=Hz.num{1}  Denominator=Hz.den{1}  SampleTime=-1  StateDataTypeStr=fixdt(1,64,29)  NumCoefDataTypeStr=fixdt(1,64,39)  DenCoefDataTypeStr=fixdt(1,64,29)  NumProductDataTypeStr=fixdt(1,64,39)  DenProductDataTypeStr=fixdt(1,64,29)  NumAccumDataTypeStr=fixdt(1,64,35)  DenAccumDataTypeStr=fixdt(1,64,25)  OutDataTypeStr=fixdt(1,64,20)  RndMeth=Nearest  SaturateOnIntegerOverflow=on
  Discrete Transfer Fcn5 : DiscreteTransferFcn  Numerator=Hz.num{1}  Denominator=Hz.den{1}  SampleTime=-1  StateDataTypeStr=fixdt(1,64,29)  NumCoefDataTypeStr=fixdt(1,64,39)  DenCoefDataTypeStr=fixdt(1,64,29)  NumProductDataTypeStr=fixdt(1,64,39)  DenProductDataTypeStr=fixdt(1,64,29)  NumAccumDataTypeStr=fixdt(1,64,35)  DenAccumDataTypeStr=fixdt(1,64,25)  OutDataTypeStr=fixdt(1,64,20)  RndMeth=Nearest  SaturateOnIntegerOverflow=on
  Mux : Mux  Inputs=3
  Unit Delay : UnitDelay  SampleTime=-1
  limit_rate_subsys : Subsystem
  Xr_set : Outport
  wires:
  Xe_set/1 -> Demux/1
  Mux/1 -> limit_rate_subsys/1(Xd)
  limit_rate_subsys/1(Xr) -> Xr_set/1, Unit Delay/1
  Unit Delay/1 -> limit_rate_subsys/2(Xd_prev)
  Constant/1 -> limit_rate_subsys/3(Tsamp)
  Constant1/1 -> limit_rate_subsys/4(Vmax)
  Demux/1 -> Discrete Transfer Fcn3/1
  Discrete Transfer Fcn3/1 -> DTC/1
  Demux/2 -> Discrete Transfer Fcn4/1
  Discrete Transfer Fcn4/1 -> DTC1/1
  Demux/3 -> Discrete Transfer Fcn5/1
  Discrete Transfer Fcn5/1 -> DTC2/1
  DTC/1 -> Mux/1
  DTC1/1 -> Mux/2
  DTC2/1 -> Mux/3

== system Quadrotor_14_step4_disc/Quadrotor/Subsystem/Outer_Loop/sensor_fusion ==
  Xe_f : Inport
  Ve_f : Inport  Port=2
  Xe_s : Inport  Port=3
  Ve_s : Inport  Port=4
  Subsystem : Subsystem
  anti-aliasing : Subsystem  mask{tau=tau, Ts=Ts}
      mask prompts: tau "tau (sec)"; Ts "Ts (sec)"
      mask init:
      | Hs = tf(1,[tau,1]);
      | Hz = ipesh_transform(Hs,Ts);
  Xe : Outport
  Ve : Outport  Port=2
  wires:
  anti-aliasing/1(y) -> Xe/1
  Subsystem/1(Xe) -> anti-aliasing/1(u)
  Subsystem/2(Ve) -> Ve/1
  Xe_f/1 -> Subsystem/1(Xe_f)
  Ve_f/1 -> Subsystem/2(Ve_f)
  Ve_s/1 -> Subsystem/3(Ve_s)
  Xe_s/1 -> Subsystem/4(Xe_s)

== system Quadrotor_14_step4_disc/Quadrotor/Subsystem/sensor_convert/lat_long_to_XY_subsys ==
  lat : Inport
  lon : Inport  Port=2
  DTC{,1..6,27} (8 alike) : DataTypeConversion
  Mux : Mux  Inputs=2
  Product : Product  OutDataTypeStr=fixdt(1,32,24)  RndMeth=Zero
  Product1 : Product  OutDataTypeStr=fixdt(1,32,24)  RndMeth=Zero
  Sum : Sum  Inputs=+-|  OutDataTypeStr=fixdt(1,32,47)
  Sum1 : Sum  Inputs=+-|  OutDataTypeStr=fixdt(1,32,46)
  TF1 : simulink/Lookup Tables/Sine  SystemSampleTime=-1  Formula=sin(2*pi*u)  NumDataPoints=(2^7)+1  OutputWordLength=32
  TF6 : simulink/Lookup Tables/Cosine  SystemSampleTime=-1  Formula=cos(2*pi*u)  NumDataPoints=(2^7)+1  OutputWordLength=32
  angle : Subsystem
  dist : Subsystem
  lat_lon_0 : Subsystem
  rescale : Gain  Gain=1/(2*pi)  ParamMin=1/(2*pi)  ParamMax=1/(2*pi)  OutDataTypeStr=fixdt(1,32,33)
  rescale1 : Gain  Gain=1/(2*pi)  ParamMin=1/(2*pi)  ParamMax=1/(2*pi)  OutDataTypeStr=fixdt(1,32,33)
  to_rads : Gain  Gain=pi/180e7  ParamMin=pi/180e7  ParamMax=pi/180e7  OutDataTypeStr=fixdt(1,32,31)
  to_rads1 : Gain  Gain=pi/180e7  ParamMin=pi/180e7  ParamMax=pi/180e7  OutDataTypeStr=fixdt(1,32,30)
  XY : Outport
  wires:
  to_rads/1 -> DTC/1  "lat"
  to_rads1/1 -> DTC1/1  "lon"
  lat_lon_0/1(lat_0) -> Sum/2, angle/2(lat_0)
  lat_lon_0/2(lon_0) -> Sum1/2
  Sum/1 -> dist/1(del_lat)
  Sum1/1 -> dist/2(del_lon), angle/3(del_lon)
  angle/1(theta) -> rescale/1, rescale1/1
  TF6/1 -> DTC6/1
  TF1/1 -> DTC5/1
  dist/1(d) -> Product/2, Product1/2
  Product/1 -> DTC2/1
  Product1/1 -> DTC3/1
  lat/1 -> to_rads/1
  lon/1 -> to_rads1/1
  Mux/1 -> XY/1
  DTC/1 -> lat_lon_0/1(lat), angle/1(lat), Sum/1, dist/3(lat)
  DTC1/1 -> lat_lon_0/2(lon), Sum1/1
  DTC2/1 -> Mux/1
  DTC3/1 -> Mux/2
  rescale/1 -> DTC27/1
  DTC27/1 -> TF6/1
  rescale1/1 -> DTC4/1
  DTC4/1 -> TF1/1
  DTC5/1 -> Product1/1
  DTC6/1 -> Product/1

== system Quadrotor_14_step4_disc/Quadrotor/Subsystem/sensor_convert/match_yaw_subsys ==
  u : Inport
  Constant : Constant  Value=360  OutMin=360  OutMax=360  OutDataTypeStr=fixdt(1,32,22)
  Data Type Conversion : DataTypeConversion
  Sum : Sum  Inputs=+-|  OutDataTypeStr=fixdt(1,32,18)
  Switch : Switch  Criteria=u2 > Threshold  Threshold=180 * 100  OutDataTypeStr=fixdt(1,32,16)
  euler_gain1 : Gain  Gain=100  ParamMin=100  ParamMax=100  OutDataTypeStr=fixdt(1,32,15)
  y : Outport
  wires:
  u/1 -> Sum/1, Switch/2, Switch/3
  Constant/1 -> euler_gain1/1
  euler_gain1/1 -> Data Type Conversion/1
  Switch/1 -> y/1
  Sum/1 -> Switch/1
  Data Type Conversion/1 -> Sum/2

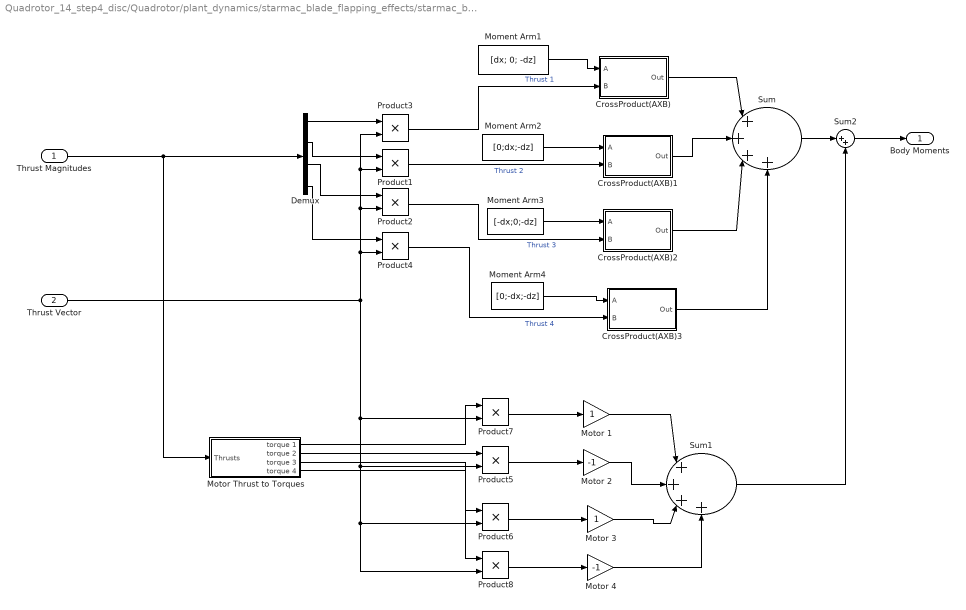
== system Quadrotor_14_step4_disc/Quadrotor/plant_dynamics/starmac_blade_flapping_effects/starmac_body_moments ==
  Thrust Magnitudes : Inport
  Thrust Vector : Inport  Port=2
  CrossProduct(AXB) : Subsystem
  CrossProduct(AXB)1 : Subsystem
  CrossProduct(AXB)2 : Subsystem
  CrossProduct(AXB)3 : Subsystem
  Demux : Demux
  Moment Arm1 : Constant  Value=[dx; 0; -dz]
  Moment Arm2 : Constant  Value=[0;dx;-dz]
  Moment Arm3 : Constant  Value=[-dx;0;-dz]
  Moment Arm4 : Constant  Value=[0;-dx;-dz]
  Motor 1 : Gain
  Motor 2 : Gain  Gain=-1
  Motor 3 : Gain
  Motor 4 : Gain  Gain=-1
  Motor Thrust to Torques : Subsystem
  Product{1..8} (8 alike) : Product  RndMeth=Zero
  Sum : Sum  Inputs=|++++
  Sum1 : Sum  Inputs=|++++
  Sum2 : Sum  Inputs=|++
  Body Moments : Outport
  wires:
  CrossProduct(AXB)1/1(Out) -> Sum/2
  Motor Thrust to Torques/4(torque 4) -> Product8/1
  Motor Thrust to Torques/3(torque 3) -> Product6/1
  Motor Thrust to Torques/2(torque 2) -> Product5/1
  Motor Thrust to Torques/1(torque 1) -> Product7/1
  Product8/1 -> Motor 4/1
  Product6/1 -> Motor 3/1
  Product5/1 -> Motor 2/1
  Product7/1 -> Motor 1/1
  Sum2/1 -> Body Moments/1
  Sum1/1 -> Sum2/2
  Sum/1 -> Sum2/1
  Motor 4/1 -> Sum1/4
  Motor 3/1 -> Sum1/3
  Motor 2/1 -> Sum1/2
  Motor 1/1 -> Sum1/1
  CrossProduct(AXB)3/1(Out) -> Sum/4
  CrossProduct(AXB)2/1(Out) -> Sum/3
  CrossProduct(AXB)/1(Out) -> Sum/1
  Product4/1 -> CrossProduct(AXB)3/2(B)  "Thrust 4"
  Moment Arm4/1 -> CrossProduct(AXB)3/1(A)
  Product2/1 -> CrossProduct(AXB)2/2(B)  "Thrust 3"
  Moment Arm3/1 -> CrossProduct(AXB)2/1(A)
  Product1/1 -> CrossProduct(AXB)1/2(B)  "Thrust 2"
  Moment Arm2/1 -> CrossProduct(AXB)1/1(A)
  Product3/1 -> CrossProduct(AXB)/2(B)  "Thrust 1"
  Moment Arm1/1 -> CrossProduct(AXB)/1(A)
  Thrust Vector/1 -> Product8/2, Product6/2, Product5/2, Product7/2, Product4/2, Product2/2, Product1/2, Product3/2
  Demux/4 -> Product4/1
  Demux/3 -> Product2/1
  Demux/2 -> Product1/1
  Demux/1 -> Product3/1
  Thrust Magnitudes/1 -> Motor Thrust to Torques/1(Thrusts), Demux/1

== system Quadrotor_14_step4_disc/Quadrotor/plant_dynamics/starmac_blade_flapping_effects/starmac_flapping_dynamics ==
  Vb2_hat : Inport
  "Body Z " : Constant  Value=[0; 0; -1];
  Constant : Constant
  Divide : Product  Inputs=*/
  Dot Product : DotProduct  InputSameDT=on  OutDataTypeStr=Inherit: Inherit via internal rule
  Flap Angle Gain : Gain  Gain=K_a1s
  Gain : Gain  Gain=-1
  Gain1 : Gain  Gain=K_beta
  Gain2 : Gain  Gain=4
  Math Function : Math  Operator=sqrt  SaturateOnIntegerOverflow=on
  Product{1..4} (4 alike) : Product  RndMeth=Zero
  Sum : Sum  Inputs=|++
  Sum1 : Sum  Inputs=|++
  Trigonometric Function : Trigonometry
  Trigonometric Function1 : Trigonometry  Operator=cos
  minor_offset : Constant  Value=.001
  rotate 90 degrees : Gain  Gain=[0 -1 0;1 0 0;0 0 1]  Multiplication=Matrix(K*u)
  thrust_vector : Outport
  rotor_blade_moments : Outport  Port=2
  wires:
  minor_offset/1 -> Sum1/2
  Sum1/1 -> Divide/2
  Divide/1 -> rotate 90 degrees/1, Gain/1  "unit vector"
  Product4/1 -> Trigonometric Function1/1, Trigonometric Function/1, Gain1/1  "flap angle"
  Vb2_hat/1 -> Divide/1, Dot Product/1, Dot Product/2
  Dot Product/1 -> Math Function/1
  Math Function/1 -> Sum1/1, Flap Angle Gain/1  "v"
  Trigonometric Function1/1 -> Product1/2
  Trigonometric Function/1 -> Product3/1
  Product3/1 -> Sum/2
  Gain/1 -> Product3/2
  Product1/1 -> Sum/1
  "Body Z "/1 -> Product1/1
  Sum/1 -> thrust_vector/1
  Gain2/1 -> rotor_blade_moments/1
  Product2/1 -> Gain2/1
  rotate 90 degrees/1 -> Product2/2
  Gain1/1 -> Product2/1
  Flap Angle Gain/1 -> Product4/2
  Constant/1 -> Product4/1

== system Quadrotor_14_step4_disc/Quadrotor/plant_dynamics/starmac_blade_flapping_effects/starmac_vertical_effect_dynamics ==
  motor_thrusts : Inport
  v_body_relative : Inport  Port=2
  Demux : Demux
  Mux : Mux
  starmac_motor_vertical_effect_dynamics{,1..3} (4 alike) : aero_sim_lib/starmac_motor_vertical_effect_dynamics  SystemSampleTime=-1  tau_motor=tau_motor  R=R  Alpha=Alpha  Vinf=Vinf  Vh=Vh  ToverTh=ToverTh
  thrust_multiplier : Outport
  wires:
  motor_thrusts/1 -> Demux/1
  Mux/1 -> thrust_multiplier/1
  Demux/1 -> starmac_motor_vertical_effect_dynamics/1
  Demux/2 -> starmac_motor_vertical_effect_dynamics1/1
  Demux/3 -> starmac_motor_vertical_effect_dynamics2/1
  Demux/4 -> starmac_motor_vertical_effect_dynamics3/1
  starmac_motor_vertical_effect_dynamics/1 -> Mux/1
  starmac_motor_vertical_effect_dynamics1/1 -> Mux/2
  starmac_motor_vertical_effect_dynamics2/1 -> Mux/3
  starmac_motor_vertical_effect_dynamics3/1 -> Mux/4
  v_body_relative/1 -> starmac_motor_vertical_effect_dynamics2/2, starmac_motor_vertical_effect_dynamics3/2, starmac_motor_vertical_effect_dynamics1/2, starmac_motor_vertical_effect_dynamics/2

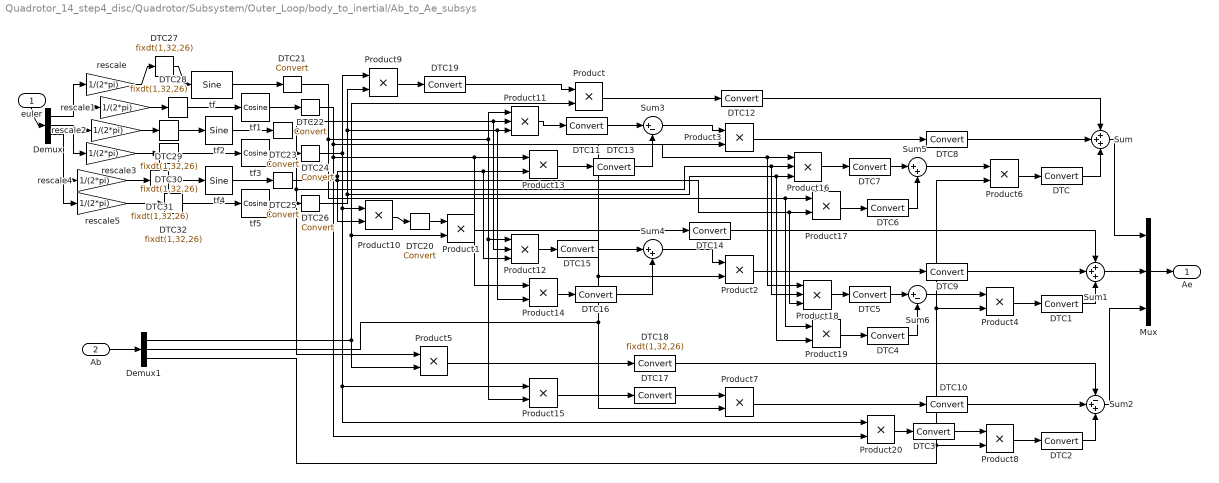
== system Quadrotor_14_step4_disc/Quadrotor/Subsystem/Outer_Loop/body_to_inertial/Ab_to_Ae_subsys ==
  euler : Inport
  Ab : Inport  Port=2
  DTC{,1..17,19..26} (26 alike) : DataTypeConversion
  DTC{18,27..32} (7 alike) : DataTypeConversion  OutDataTypeStr=fixdt(1,32,26)
  Demux : Demux  Outputs=3
  Demux1 : Demux  Outputs=3
  Mux : Mux  Inputs=3
  Product : Product  OutDataTypeStr=fixdt(1,32,33)  RndMeth=Zero
  Product1 : Product  OutDataTypeStr=fixdt(1,32,34)  RndMeth=Zero
  Product{5,9..10,15} (4 alike) : Product  OutDataTypeStr=fixdt(1,64,52)  RndMeth=Zero
  Product11 : Product  Inputs=3  OutDataTypeStr=fixdt(1,64,52)  RndMeth=Zero
  Product12 : Product  Inputs=3  OutDataTypeStr=fixdt(1,32,41)  RndMeth=Zero
  Product13 : Product  OutDataTypeStr=fixdt(1,32,31)  RndMeth=Zero
  Product14 : Product  OutDataTypeStr=fixdt(1,32,30)  RndMeth=Zero
  Product16 : Product  Inputs=3  OutDataTypeStr=fixdt(1,32,35)  RndMeth=Zero
  Product17 : Product  OutDataTypeStr=fixdt(1,32,36)  RndMeth=Zero
  Product18 : Product  Inputs=3  OutDataTypeStr=fixdt(1,32,35)  RndMeth=Zero
  Product19 : Product  OutDataTypeStr=fixdt(1,32,35)  RndMeth=Zero
  Product2 : Product  OutDataTypeStr=fixdt(1,32,33)  RndMeth=Zero
  Product20 : Product  OutDataTypeStr=fixdt(1,32,30)  RndMeth=Zero
  Product3 : Product  OutDataTypeStr=fixdt(1,32,34)  RndMeth=Zero
  Product4 : Product  OutDataTypeStr=fixdt(1,32,39)  RndMeth=Zero
  Product6 : Product  OutDataTypeStr=fixdt(1,32,39)  RndMeth=Zero
  Product7 : Product  OutDataTypeStr=fixdt(1,32,38)  RndMeth=Zero
  Product8 : Product  OutDataTypeStr=fixdt(1,32,30)  RndMeth=Zero
  Sum : Sum  Inputs=+++  OutDataTypeStr=fixdt(1,32,30)
  Sum1 : Sum  Inputs=+++  OutDataTypeStr=fixdt(1,32,30)
  Sum2 : Sum  Inputs=-++  OutDataTypeStr=fixdt(1,32,30)
  Sum3 : Sum  Inputs=|+-  OutDataTypeStr=fixdt(1,32,31)
  Sum4 : Sum  Inputs=|++  OutDataTypeStr=fixdt(1,32,30)
  Sum5 : Sum  Inputs=|++  OutDataTypeStr=fixdt(1,32,36)
  Sum6 : Sum  Inputs=|+-  OutDataTypeStr=fixdt(1,32,35)
  rescale{,1..5} (6 alike) : Gain  Gain=1/(2*pi)  ParamMin=1/(2*pi)  ParamMax=1/(2*pi)  OutDataTypeStr=fixdt(1,64,58)
  tf : simulink/Lookup Tables/Sine  SystemSampleTime=-1  Formula=sin(2*pi*u)  NumDataPoints=(2^7)+1  OutputWordLength=32
  tf1 : simulink/Lookup Tables/Cosine  SystemSampleTime=-1  Formula=cos(2*pi*u)  NumDataPoints=(2^7)+1  OutputWordLength=32
  tf2 : simulink/Lookup Tables/Sine  SystemSampleTime=-1  Formula=sin(2*pi*u)  NumDataPoints=(2^7)+1  OutputWordLength=32
  tf3 : simulink/Lookup Tables/Cosine  SystemSampleTime=-1  Formula=cos(2*pi*u)  NumDataPoints=(2^7)+1  OutputWordLength=32
  tf4 : simulink/Lookup Tables/Sine  SystemSampleTime=-1  Formula=sin(2*pi*u)  NumDataPoints=(2^7)+1  OutputWordLength=32
  tf5 : simulink/Lookup Tables/Cosine  SystemSampleTime=-1  Formula=cos(2*pi*u)  NumDataPoints=(2^7)+1  OutputWordLength=32
  Ae : Outport
  wires:
  Demux/1 -> rescale/1, rescale1/1
  Demux/2 -> rescale2/1, rescale3/1
  Demux/3 -> rescale4/1, rescale5/1
  Product/1 -> DTC12/1
  Product3/1 -> DTC8/1
  Product6/1 -> DTC/1
  Product1/1 -> DTC14/1
  Product2/1 -> DTC9/1
  Product4/1 -> DTC1/1
  Product5/1 -> DTC18/1
  Product7/1 -> DTC10/1
  Product8/1 -> DTC2/1
  tf3/1 -> DTC24/1
  tf5/1 -> DTC26/1
  Product9/1 -> DTC19/1
  Demux1/1 -> Product/2, Product1/2, Product5/2
  tf4/1 -> DTC25/1
  Product10/1 -> DTC20/1
  tf2/1 -> DTC23/1
  Product11/1 -> DTC11/1
  tf/1 -> DTC21/1
  tf1/1 -> DTC22/1
  Product13/1 -> DTC13/1
  Sum3/1 -> Product3/1
  Demux1/2 -> Product3/2, Product2/2, Product7/2
  Product12/1 -> DTC15/1
  Product14/1 -> DTC16/1
  Sum4/1 -> Product2/1
  Product15/1 -> DTC17/1
  Product16/1 -> DTC7/1
  Product17/1 -> DTC6/1
  Product18/1 -> DTC5/1
  Product19/1 -> DTC4/1
  Sum5/1 -> Product6/1
  Sum6/1 -> Product4/1
  Product20/1 -> DTC3/1
  Demux1/3 -> Product8/2, Product4/2, Product6/2
  Sum/1 -> Mux/1
  Sum1/1 -> Mux/2
  Sum2/1 -> Mux/3
  euler/1 -> Demux/1
  Ab/1 -> Demux1/1
  Mux/1 -> Ae/1
  DTC/1 -> Sum/3
  DTC1/1 -> Sum1/3
  DTC2/1 -> Sum2/3
  DTC3/1 -> Product8/1
  DTC4/1 -> Sum6/2
  DTC5/1 -> Sum6/1
  DTC6/1 -> Sum5/2
  DTC7/1 -> Sum5/1
  DTC8/1 -> Sum/2
  DTC9/1 -> Sum1/2
  DTC10/1 -> Sum2/2
  DTC11/1 -> Sum3/1
  DTC12/1 -> Sum/1
  DTC13/1 -> Sum3/2
  DTC14/1 -> Sum1/1
  DTC15/1 -> Sum4/1
  DTC16/1 -> Sum4/2
  DTC17/1 -> Product7/1
  DTC18/1 -> Sum2/1
  DTC19/1 -> Product/1
  DTC20/1 -> Product1/1
  DTC21/1 -> Product11/1, Product12/1, Product15/2, Product17/1, Product19/1
  DTC22/1 -> Product16/1, Product18/1, Product13/1, Product14/1, Product20/2
  DTC23/1 -> Product11/2, Product12/2, Product5/1, Product16/2, Product18/2
  DTC24/1 -> Product9/1, Product10/1, Product15/1, Product20/1
  DTC25/1 -> Product10/2, Product13/2, Product12/3, Product17/2, Product18/3
  DTC26/1 -> Product9/2, Product11/3, Product14/2, Product16/3, Product19/2
  rescale/1 -> DTC27/1
  DTC27/1 -> tf/1
  rescale1/1 -> DTC28/1
  DTC28/1 -> tf1/1
  rescale2/1 -> DTC29/1
  DTC29/1 -> tf2/1
  rescale3/1 -> DTC30/1
  DTC30/1 -> tf3/1
  rescale4/1 -> DTC31/1
  DTC31/1 -> tf4/1
  rescale5/1 -> DTC32/1
  DTC32/1 -> tf5/1
